simulink model "TD2"  (R2017b)
settings: Solver=ode15s  StartTime=0.0  StopTime=5  RelTol=1e-3
values from neighbouring files (symbols this model uses):
  b = 3.5077e-6    (= 3.5077e-06)    [MCC_variables.m]    (also in TD2_config.m = 0.0085)
  J = 3.2284e-6    (= 3.2284e-06)    [MCC_variables.m]    (also in TD2_config.m = 0.28; TD3.m = 0.2)
  K = 0.0274    [MCC_variables.m]    (also in TD2_config.m = 0.5093; TD3.m = 0.9)
  Kd = 0.2    [TD2_config.m]
  Ki = 140    [TD2_config.m]
  Kp = 20    [TD2_config.m]
  Kpos = 1    [TD2_config.m]
  L = 2.75e-6    (= 2.75e-06)    [MCC_variables.m]    (also in TD2_config.m = 0.0016)
  R = 4    [MCC_variables.m]    (also in TD2_config.m = 0.13; TD3.m = 0.895)
libraries: simulink x1
settings Model: Creator=Table2  LastModifiedBy=Table2

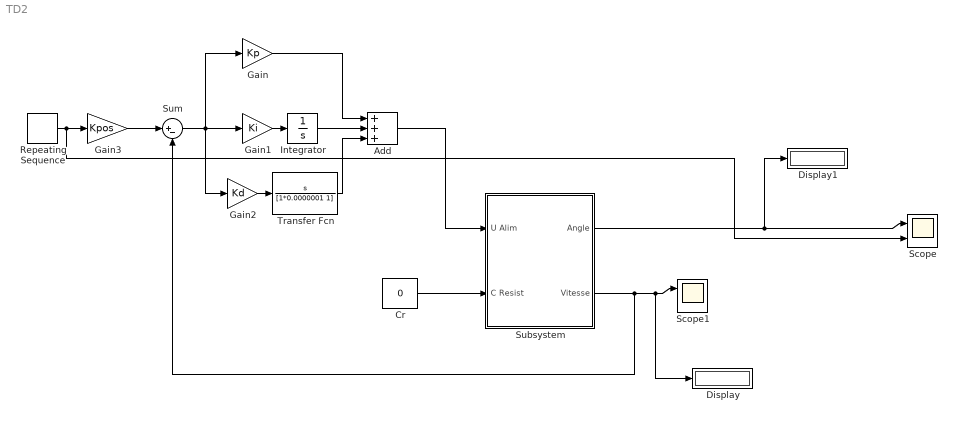
== system TD2 ==
  Add : Sum  Inputs=+++
  Cr : Constant  Value=0
  Display : Display
  Display1 : Display
  Gain : Gain  Gain=Kp
  Gain1 : Gain  Gain=Ki
  Gain2 : Gain  Gain=Kd
  Gain3 : Gain  Gain=Kpos
  Integrator : Integrator
  Repeating Sequence : simulink/Sources/Repeating Sequence  rep_seq_t=[0 0.1 0.2 0.3 1]  rep_seq_y=[0 50 50 0 0]
  Scope : Scope  NumInputPorts=2
  Scope1 : Scope  NumInputPorts=2
  Subsystem : Subsystem
  Sum : Sum  Inputs=|+-
  Transfer Fcn : TransferFcn  Numerator=[1 0]  Denominator=[1*0.0000001 1]
  wires:
  Cr/1 -> Subsystem/2(C Resist)
  Subsystem/1(Angle) -> Display1/1, Scope/1
  Subsystem/2(Vitesse) -> Sum/2, Display/1, Scope1/1
  Add/1 -> Subsystem/1(U Alim)
  Gain/1 -> Add/1
  Gain1/1 -> Integrator/1
  Integrator/1 -> Add/2
  Sum/1 -> Gain2/1, Gain1/1, Gain/1
  Gain2/1 -> Transfer Fcn/1
  Transfer Fcn/1 -> Add/3
  Gain3/1 -> Sum/1
  Repeating Sequence/1 -> Scope/2, Gain3/1

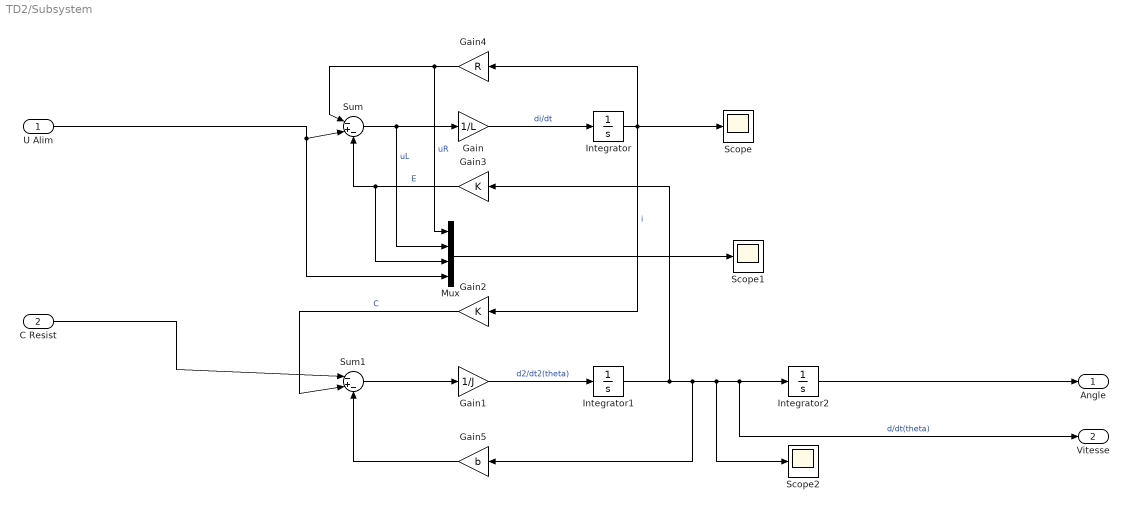
== system TD2/Subsystem ==
  U Alim : Inport
  C Resist : Inport  Port=2
  Gain : Gain  Gain=1/L
  Gain1 : Gain  Gain=1/J
  Gain2 : Gain  Gain=K
  Gain3 : Gain  Gain=K
  Gain4 : Gain  Gain=R
  Gain5 : Gain  Gain=b
  Integrator : Integrator
  Integrator1 : Integrator
  Integrator2 : Integrator
  Mux : Mux
  Scope : Scope
  Scope1 : Scope
  Scope2 : Scope
  Sum : Sum  Inputs=|-+-
  Sum1 : Sum  Inputs=|-+-
  Angle : Outport
  Vitesse : Outport  Port=2
  wires:
  Integrator/1 -> Gain2/1, Scope/1, Gain4/1  "i"
  Gain2/1 -> Sum1/2  "C"
  Integrator1/1 -> Gain3/1, Gain5/1, Scope2/1, Vitesse/1, Integrator2/1  "d/dt(theta)"
  Gain1/1 -> Integrator1/1  "d2/dt2(theta)"
  Sum1/1 -> Gain1/1
  Gain3/1 -> Mux/3, Sum/3  "E"
  U Alim/1 -> Mux/4, Sum/2
  Gain4/1 -> Mux/1, Sum/1  "uR"
  C Resist/1 -> Sum1/1
  Gain/1 -> Integrator/1  "di/dt"
  Sum/1 -> Mux/2, Gain/1  "uL"
  Gain5/1 -> Sum1/3
  Integrator2/1 -> Angle/1
  Mux/1 -> Scope1/1
